simulink model "DestinationControl"  (R2020a)
settings: Solver=ode3  StartTime=0.0  StopTime=10.0  RelTol=1e-3
PreLoadFcn:
  | % Lidar parameters
  | 
  | scanAngles = linspace(-pi/2,pi/2,360);
  | scanMaxRange = 3.5;
  | scanSensorOffset = [0,0];
undefined symbols (not defined in the file or in its folder): Angular, Linear
libraries: robotlib x5, robotalgslib x1
settings Model: Creator=Pierre  LastModifiedBy=Pierre
settings OptimizationCC: EnhancedBackFolding=on  PassReuseOutputArgsAs=Individual arguments  ZeroExternalMemoryAtStartup=off  ZeroInternalMemoryAtStartup=off  MaxStackSize=64  OptimizeBlockOrder=speed  DifferentSizesBufferReuse=on  OptimizationCustomize=off  EfficientTunableParamExpr=on
settings DebuggingCC: ParameterTunabilityLossMsg=error
settings HardwareCC: ProdBitPerPointer=32  ProdBitPerSizeT=32  ProdBitPerPtrDiffT=32  ProdLargestAtomicFloat=None  ProdIntDivRoundTo=Undefined  ProdEndianess=Unspecified  ProdWordSize=32  ProdHWDeviceType=Generic->Unspecified (assume 32-bit Generic)
settings SFSimCC: MATLABDynamicMemAlloc=off
settings RTWCC: SystemTargetFile=ert.tlc  HardwareBoard=Robot Operating System (ROS)  TemplateMakefile=ert_default_tmf  Toolchain=Catkin  TargetLang=C++
settings CodeAppCC: ForceParamTrailComments=on  IgnoreCustomStorageClasses=off  OperatorAnnotations=on  SimulinkDataObjDesc=on  SFDataObjDesc=on  InsertBlockDesc=on
settings ERTTargetCC: SupportVariableSizeSignals=on

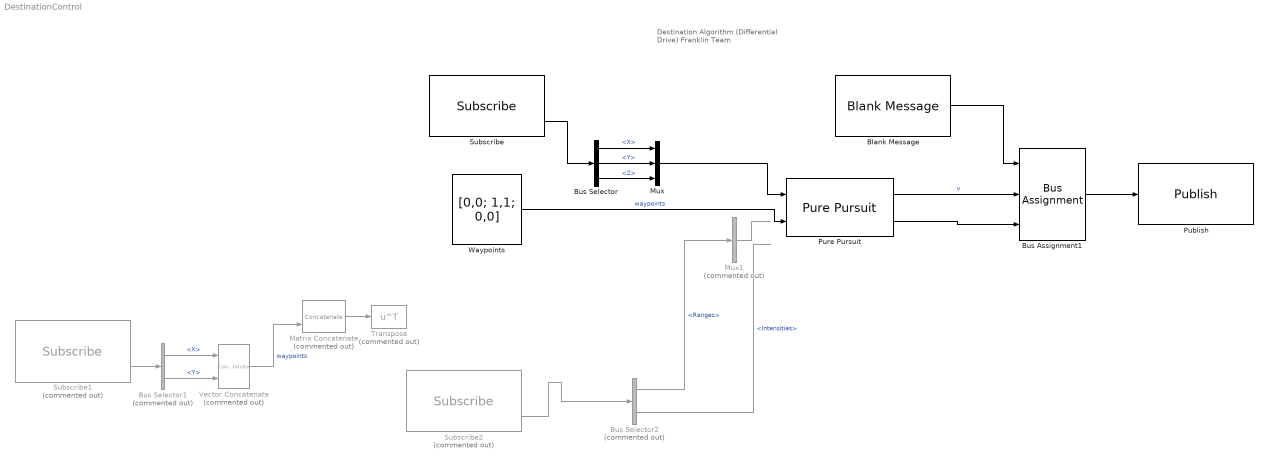
== system DestinationControl ==
  note: Destination Algorithm
      | (Differential Drive)
      |
      | Franklin Team
  Blank Message : robotlib/Blank Message  messageClass=Message  entityType=geometry_msgs/Twist  messageType=geometry_msgs/Twist  SampleTime=inf
  Bus Assignment1 : BusAssignment  AssignedSignals=Linear.X,Angular.Z
  Bus Selector : BusSelector  OutputSignals=Pose.Pose.Position.X,Pose.Pose.Position.Y,Pose.Pose.Orientation.Z
  Bus Selector1 : BusSelector  Commented=on  OutputSignals=X,Y
  Bus Selector2 : BusSelector  Commented=on  OutputSignals=Ranges,Intensities
  Matrix Concatenate : Concatenate  Commented=on  Mode=Multidimensional array  ConcatenateDimension=2
  Mux : Mux  Inputs=3
  Mux1 : Mux  Commented=on  Inputs=1
  Publish : robotlib/Publish  topicSource=Specify your own  topic=/cmd_vel  messageType=geometry_msgs/Twist  messageQueueLength=1
  Pure Pursuit : robotalgslib/Pure Pursuit  DesiredLinearVelocity=0.1  MaxAngularVelocity=1.0  LookaheadDistance=1.0  TargetDirPort=off  SimulateUsing=Code generation
  Subscribe : robotlib/Subscribe  topicSource=Specify your own  topic=/odom  messageType=nav_msgs/Odometry  sampleTime=-1  messageQueueLength=1
  Subscribe1 : robotlib/Subscribe  Commented=on  topicSource=Specify your own  topic=/destination  messageType=geometry_msgs/Point  sampleTime=-1  messageQueueLength=1
  Subscribe2 : robotlib/Subscribe  Commented=on  topicSource=Specify your own  topic=/scan  messageType=sensor_msgs/LaserScan  sampleTime=-1  messageQueueLength=1
  Transpose : Math  Commented=on  Operator=transpose  SignedPower=on  RndMeth=Zero  SaturateOnIntegerOverflow=on
  Vector Concatenate : Concatenate  Commented=on  ConcatenateDimension=2
  Waypoints : Constant  Value=[0,0; 1,1; 0,0]
  wires:
  Subscribe/2 -> Bus Selector/1
  Blank Message/1 -> Bus Assignment1/1
  Bus Selector/1 -> Mux/1  "<X>"
  Bus Selector/2 -> Mux/2  "<Y>"
  Bus Selector/3 -> Mux/3  "<Z>"
  Subscribe1/2 -> Bus Selector1/1
  Bus Selector1/1 -> Vector Concatenate/1  "<X>"
  Bus Selector1/2 -> Vector Concatenate/2  "<Y>"
  Matrix Concatenate/1 -> Transpose/1
  Vector Concatenate/1 -> Matrix Concatenate/2  "waypoints"
  Bus Assignment1/1 -> Publish/1
  Pure Pursuit/1 -> Bus Assignment1/2  "v"
  Mux/1 -> Pure Pursuit/1
  Waypoints/1 -> Pure Pursuit/2  "waypoints"
  Subscribe2/2 -> Bus Selector2/1
  Bus Selector2/1 -> Mux1/1  "<Ranges>"
  Mux1/1 -> ?
  Bus Selector2/2 -> ?  "<Intensities>"
  Pure Pursuit/2 -> Bus Assignment1/3
